simulink model "Full_RC_EVOP"  (Simulink 9.2)
settings: Solver=ode3  StartTime=0.0  StopTime=50000.0  FixedStep=0.01  RelTol=1e-3  EnableMultiTasking=on
settings Model: Creator=user  LastModifiedBy=user
settings DataIOCC: SignalLoggingSaveFormat=Dataset
settings DebuggingCC: UnderspecifiedInitializationDetection=Simplified  MergeDetectMultiDrivingBlocksExec=error  SolverPrmCheckMsg=warning  FcnCallInpInsideContextMsg=error  StateNameClashWarn=none
settings GRTTargetCC: CombineOutputUpdateFcns=on  GRTInterface=off
settings ConfigComp: CovSFcnEnable=off

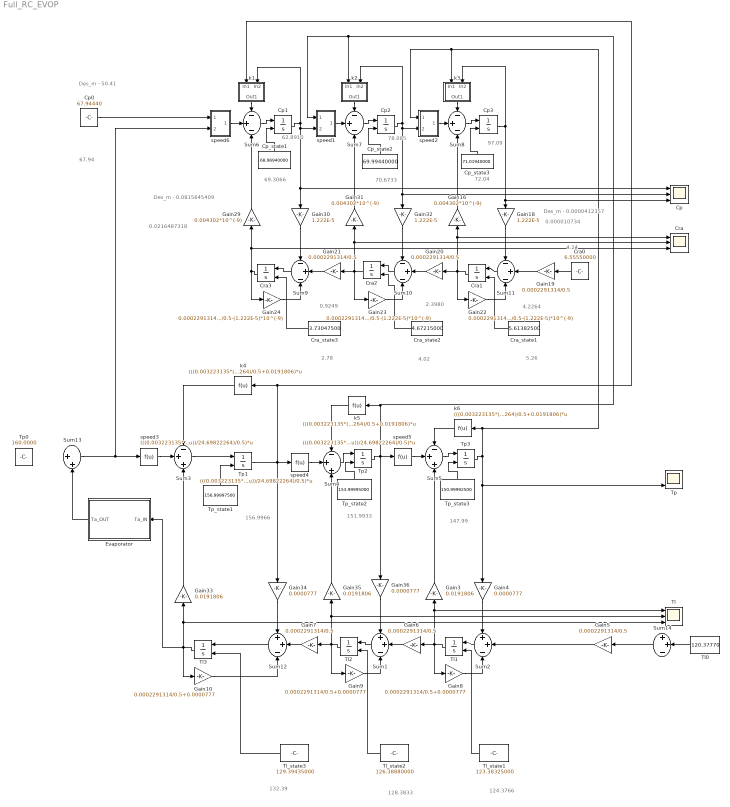
== system Full_RC_EVOP ==
  note: Des_m - 0.0000412357
  note: Des_m - 0.0815645409
  note: 0.000010734
  note: 0.0216487318
  note: 0.9249
  note: 2.3980
  note: 4.2264
  note: 62.8910
  note: 78.085
  note: 97.09
  note: 67.94
  note: 2.78
  note: 4.02
  note: 5.26
  note: 72.04
  note: 70.6733
  note: 69.3066
  note: 132.39
  note: 128.3833
  note: 124.3766
  note: 147.99
  note: 151.9933
  note: 156.9966
  note: 4.24
  note: Des_m - 50.41
  Cp : Scope  NumInputPorts=3
  Cp0 : Constant  Value=67.94440
  Cp1 : Integrator  InitialConditionSource=external  InitialCondition=69.3066
  Cp2 : Integrator  InitialConditionSource=external  InitialCondition=70.6733
  Cp3 : Integrator  InitialConditionSource=external  InitialCondition=72.04
  Cp_state1 : Constant  Value=68.96940000
  Cp_state2 : Constant  Value=69.99440000
  Cp_state3 : Constant  Value=71.01940000
  Cra : Scope  NumInputPorts=3
  Cra0 : Constant  Value=6.55550000
  Cra1 : Integrator  InitialConditionSource=external  InitialCondition=5.26
  Cra2 : Integrator  InitialConditionSource=external  InitialCondition=4.02
  Cra3 : Integrator  InitialConditionSource=external  InitialCondition=2.78
  Cra_state1 : Constant  Value=5.61382500
  Cra_state2 : Constant  Value=4.67215000
  Cra_state3 : Constant  Value=3.73047500
  Evaporator : Subsystem
  Gain10 : Gain  Gain=0.0002291314/0.5+0.0000777
  Gain16 : Gain  Gain=0.004302*10^(-9)
  Gain18 : Gain  Gain=1.222E-5
  Gain{5..7,19..21} (6 alike) : Gain  Gain=0.0002291314/0.5
  Gain22 : Gain  Gain=0.0002291314/0.5-(1.222E-5)*10^(-9)
  Gain23 : Gain  Gain=0.0002291314/0.5-(1.222E-5)*10^(-9)
  Gain24 : Gain  Gain=0.0002291314/0.5-(1.222E-5)*10^(-9)
  Gain29 : Gain  Gain=0.004302*10^(-9)
  Gain3 : Gain  Gain=0.0191806
  Gain30 : Gain  Gain=1.222E-5
  Gain31 : Gain  Gain=0.004302*10^(-9)
  Gain32 : Gain  Gain=1.222E-5
  Gain33 : Gain  Gain=0.0191806
  Gain34 : Gain  Gain=0.0000777
  Gain35 : Gain  Gain=0.0191806
  Gain36 : Gain  Gain=0.0000777
  Gain4 : Gain  Gain=0.0000777
  Gain8 : Gain  Gain=0.0002291314/0.5+0.0000777
  Gain9 : Gain  Gain=0.0002291314/0.5+0.0000777
  Sum{1..2,12,14} (4 alike) : Sum  Inputs=++-
  Sum{6..11} (6 alike) : Sum  Inputs=-+-
  Sum13 : Sum  Inputs=|++
  Sum3 : Sum  Inputs=-++
  Sum4 : Sum  Inputs=-++
  Sum5 : Sum  Inputs=-++
  Tl : Scope  NumInputPorts=3
  Tl0 : Constant  Value=120.37770
  Tl1 : Integrator  InitialConditionSource=external  InitialCondition=124.3766
  Tl2 : Integrator  InitialConditionSource=external  InitialCondition=128.3833
  Tl3 : Integrator  InitialConditionSource=external  InitialCondition=132.39
  "Tl_state1 " : Constant  Value=123.38325000
  Tl_state2 : Constant  Value=126.38880000
  Tl_state3 : Constant  Value=129.39435000
  Tp : Scope  NumInputPorts=3
  Tp0 : Constant  Value=160.0000
  Tp1 : Integrator  InitialConditionSource=external  InitialCondition=156.9966
  Tp2 : Integrator  InitialConditionSource=external  InitialCondition=151.9933
  Tp3 : Integrator  InitialConditionSource=external  InitialCondition=147.99  IgnoreLimit=on
  Tp_state1 : Constant  Value=156.99997500
  Tp_state2 : Constant  Value=153.99995000
  Tp_state3 : Constant  Value=150.99992500
  k1 : Subsystem
  k2 : Subsystem
  k3 : Subsystem
  k4 : Fcn  Expr=(((0.003223135*(273+u))/24.69822264)/0.5+0.0191806)*u
  k5 : Fcn  Expr=(((0.003223135*(273+u))/24.69822264)/0.5+0.0191806)*u
  k6 : Fcn  Expr=(((0.003223135*(273+u))/24.69822264)/0.5+0.0191806)*u
  speed1 : Subsystem
  speed2 : Subsystem
  speed3 : Fcn  Expr=(((0.003223135*(273+u))/24.69822264)/0.5)*u
  speed4 : Fcn  Expr=(((0.003223135*(273+u))/24.69822264)/0.5)*u
  speed5 : Fcn  Expr=(((0.003223135*(273+u))/24.69822264)/0.5)*u
  speed6 : Subsystem
  wires:
  Sum6/1 -> Cp1/1
  speed1/1(Out1) -> Sum7/2
  Sum7/1 -> Cp2/1
  speed2/1(Out1) -> Sum8/2
  Sum8/1 -> Cp3/1
  Cp1/1 -> speed1/2(In2), Gain30/1, Cp/1, k1/2(In2)
  Cp2/1 -> speed2/2(In2), Gain32/1, Cp/2, k2/2(In2)
  Gain29/1 -> Sum6/3
  Cp3/1 -> k3/2(In2), Gain18/1, Cp/3
  Gain31/1 -> Sum7/3
  Gain16/1 -> Sum8/3
  Gain30/1 -> Sum9/1
  Gain32/1 -> Sum10/1
  Gain18/1 -> Sum11/1
  Gain19/1 -> Sum11/2
  Sum11/1 -> Cra1/1
  Cra1/1 -> Gain22/1, Gain20/1, Gain16/1, Cra/1
  Gain20/1 -> Sum10/2
  Sum10/1 -> Cra2/1
  Cra2/1 -> Gain23/1, Gain21/1, Gain31/1, Cra/2
  Gain21/1 -> Sum9/2
  Sum9/1 -> Cra3/1
  Cra3/1 -> Gain24/1, Gain29/1, Cra/3
  Gain22/1 -> Sum11/3
  Gain23/1 -> Sum10/3
  Gain24/1 -> Sum9/3
  speed3/1 -> Sum3/2
  k4/1 -> Sum3/1
  Sum3/1 -> Tp1/1
  speed4/1 -> Sum4/2
  k5/1 -> Sum4/1
  Sum4/1 -> Tp2/1
  speed5/1 -> Sum5/2
  k6/1 -> Sum5/1
  Sum5/1 -> Tp3/1
  Gain33/1 -> Sum3/3
  Tp3/1 -> Gain4/1, Tp/3, k6/1, k3/1(In1), speed2/1(In1)
  Gain35/1 -> Sum4/3
  Gain3/1 -> Sum5/3
  Gain34/1 -> Sum12/1
  Gain36/1 -> Sum1/1
  Gain4/1 -> Sum2/1
  Gain5/1 -> Sum2/2
  Sum2/1 -> Tl1/1
  Tl1/1 -> Gain8/1, Gain6/1, Gain3/1, Tl/1
  Gain6/1 -> Sum1/2
  Sum1/1 -> Tl2/1
  Tl2/1 -> Gain9/1, Gain7/1, Gain35/1, Tl/2
  Gain7/1 -> Sum12/2
  Sum12/1 -> Tl3/1
  Tl3/1 -> Evaporator/1(Ta_IN), Gain10/1, Gain33/1, Tl/3
  Gain8/1 -> Sum2/3
  Gain9/1 -> Sum1/3
  Gain10/1 -> Sum12/3
  speed6/1(Out1) -> Sum6/2
  Cp0/1 -> speed6/1(In1)
  k1/1(Out1) -> Sum6/1
  k2/1(Out1) -> Sum7/1
  k3/1(Out1) -> Sum8/1
  Cra0/1 -> Gain19/1
  Sum13/1 -> speed3/1, speed6/2(In2)
  Sum14/1 -> Gain5/1
  Tl0/1 -> Sum14/2
  Tp2/1 -> Gain36/1, k5/1, speed1/1(In1), k2/1(In1), speed5/1
  Tp1/1 -> k4/1, k1/1(In1), Gain34/1, speed4/1
  Tp_state1/1 -> Tp1/2
  Tp_state2/1 -> Tp2/2
  Tp_state3/1 -> Tp3/2
  "Tl_state1 "/1 -> Tl1/2
  Tl_state2/1 -> Tl2/2
  Tl_state3/1 -> Tl3/2
  Cp_state1/1 -> Cp1/2
  Cp_state2/1 -> Cp2/2
  Cp_state3/1 -> Cp3/2
  Cra_state1/1 -> Cra1/2
  Cra_state2/1 -> Cra2/2
  Cra_state3/1 -> Cra3/2
  Evaporator/1(Ta_OUT) -> Sum13/2

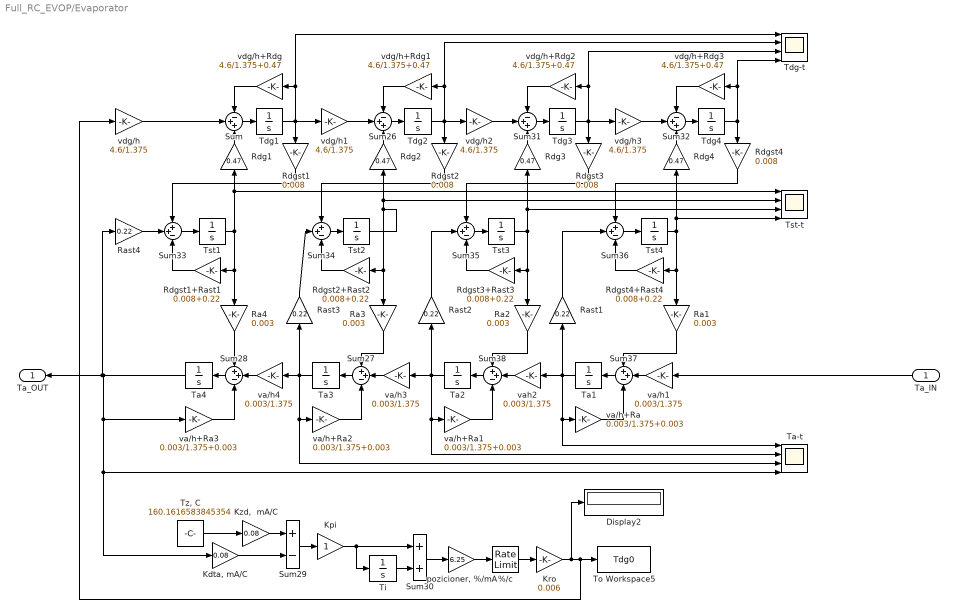
== system Full_RC_EVOP/Evaporator ==
  Ta_IN : Inport
  %/c : RateLimiter  RisingSlewLimit=5  FallingSlewLimit=-5  SampleTimeMode=inherited
  Display2 : Display
  "Kdta, mA/C" : Gain  Gain=0.08
  Kpi : Gain
  Kro : Gain  Gain=0.006
  "Kzd,  mA/C" : Gain  Gain=0.08
  Ra{1..4} (4 alike) : Gain  Gain=0.003
  Rast{1..4} (4 alike) : Gain  Gain=0.22
  Rdg{1..4} (4 alike) : Gain  Gain=0.47
  Rdgst{1..4} (4 alike) : Gain  Gain=0.008
  Rdgst1+Rast1 : Gain  Gain=0.008+0.22
  Rdgst2+Rast2 : Gain  Gain=0.008+0.22
  Rdgst3+Rast3 : Gain  Gain=0.008+0.22
  Rdgst4+Rast4 : Gain  Gain=0.008+0.22
  Sum{,26,31..32} (4 alike) : Sum  Inputs=-++
  Sum{27..28,33..38} (8 alike) : Sum  Inputs=++-
  Sum29 : Sum  Inputs=+-
  Sum30 : Sum
  Ta-t : Scope  NumInputPorts=4
  Ta1 : Integrator  InitialCondition=136.285
  Ta2 : Integrator  InitialCondition=144.19
  Ta3 : Integrator  InitialCondition=152.09
  Ta4 : Integrator  InitialCondition=160
  Tdg-t : Scope  NumInputPorts=4
  Tdg1 : Integrator  InitialCondition=283.3065209436467
  Tdg2 : Integrator  InitialCondition=267.8966165589237
  Tdg3 : Integrator  InitialCondition=253.6715917846216
  Tdg4 : Integrator  InitialCondition=240.5403403000344
  Ti : Integrator  InitialCondition=8000  UpperSaturationLimit=8012  LowerSaturationLimit=6012
  To Workspace5 : ToWorkspace  VariableName=Tdg0  SampleTime=-1
  Tst-t : Scope  NumInputPorts=4
  Tst1 : Integrator  InitialCondition=164.4825307550351
  Tst2 : Integrator  InitialCondition=158.2090959868120
  Tst3 : Integrator  InitialCondition=152.4180305285302
  Tst4 : Integrator  InitialCondition=147.0722446263660
  "Tz, C" : Constant  Value=160.1616583845354
  "pozicioner, %/mA" : Gain  Gain=6.25
  va/h+Ra{,1..3} (4 alike) : Gain  Gain=0.003/1.375+0.003
  va/h1 : Gain  Gain=0.003/1.375
  va/h3 : Gain  Gain=0.003/1.375
  va/h4 : Gain  Gain=0.003/1.375
  vah2 : Gain  Gain=0.003/1.375
  vdg/h{,1..3} (4 alike) : Gain  Gain=4.6/1.375
  vdg/h+Rdg{,1..3} (4 alike) : Gain  Gain=4.6/1.375+0.47
  Ta_OUT : Outport
  wires:
  Sum/1 -> Tdg1/1
  vdg/h2/1 -> Sum31/2
  Sum32/1 -> Tdg4/1
  Tdg2/1 -> vdg/h+Rdg1/1, Tdg-t/2, Rdgst2/1, vdg/h2/1
  Sum26/1 -> Tdg2/1
  vdg/h3/1 -> Sum32/2
  vdg/h/1 -> Sum/2
  Tdg1/1 -> vdg/h+Rdg/1, Tdg-t/1, vdg/h1/1, Rdgst1/1
  vdg/h+Rdg2/1 -> Sum31/1
  vdg/h+Rdg3/1 -> Sum32/1
  Tdg4/1 -> vdg/h+Rdg3/1, Tdg-t/4, Rdgst4/1
  Rdg1/1 -> Sum/3
  Rdg2/1 -> Sum26/3
  Rdg3/1 -> Sum31/3
  Rdg4/1 -> Sum32/3
  vdg/h+Rdg1/1 -> Sum26/1
  Sum33/1 -> Tst1/1
  Sum34/1 -> Tst2/1
  Tdg3/1 -> vdg/h+Rdg2/1, Tdg-t/3, vdg/h3/1, Rdgst3/1
  vdg/h1/1 -> Sum26/2
  Sum35/1 -> Tst3/1
  vdg/h+Rdg/1 -> Sum/1
  Sum31/1 -> Tdg3/1
  Rdgst3+Rast3/1 -> Sum35/3
  Tst1/1 -> Rdgst1+Rast1/1, Ra4/1, Rdg1/1, Tst-t/1
  Rdgst1+Rast1/1 -> Sum33/3
  Tst3/1 -> Rdgst3+Rast3/1, Ra2/1, Rdg3/1, Tst-t/3
  Tst2/1 -> Rdg2/1, Tst-t/2, Rdgst2+Rast2/1, Ra3/1
  Rdgst1/1 -> Sum33/1
  Rdgst2/1 -> Sum34/1
  Tst4/1 -> Rdgst4+Rast4/1, Ra1/1, Rdg4/1, Tst-t/4
  Rdgst4/1 -> Sum36/1
  Rdgst2+Rast2/1 -> Sum34/3
  va/h1/1 -> Sum37/2
  va/h+Ra/1 -> Sum37/3
  Rdgst3/1 -> Sum35/1
  Sum36/1 -> Tst4/1
  Rdgst4+Rast4/1 -> Sum36/3
  Ti/1 -> Sum30/2
  Ta4/1 -> Ta_OUT/1, Rast4/1, va/h+Ra3/1, Ta-t/4, "Kdta, mA/C"/1
  Rast1/1 -> Sum36/2
  Ra2/1 -> Sum38/1
  Ta2/1 -> va/h+Ra1/1, Ta-t/2, va/h3/1, Rast2/1
  va/h+Ra3/1 -> Sum28/3
  Ta1/1 -> Ta-t/1, va/h+Ra/1, Rast1/1, vah2/1
  va/h+Ra2/1 -> Sum27/3
  Rast3/1 -> Sum34/2
  Sum38/1 -> Ta2/1
  va/h4/1 -> Sum28/2
  Sum37/1 -> Ta1/1
  va/h3/1 -> Sum27/2
  Ta3/1 -> va/h+Ra2/1, Ta-t/3, va/h4/1, Rast3/1
  Rast2/1 -> Sum35/2
  "Tz, C"/1 -> "Kzd,  mA/C"/1
  "Kdta, mA/C"/1 -> Sum29/2
  %/c/1 -> Kro/1
  Ta_IN/1 -> va/h1/1
  "Kzd,  mA/C"/1 -> Sum29/1
  Sum28/1 -> Ta4/1
  Rast4/1 -> Sum33/2
  Sum27/1 -> Ta3/1
  va/h+Ra1/1 -> Sum38/3
  "pozicioner, %/mA"/1 -> %/c/1
  Ra3/1 -> Sum27/1
  Sum29/1 -> Kpi/1
  Kpi/1 -> Sum30/1, Ti/1
  Ra4/1 -> Sum28/1
  Sum30/1 -> "pozicioner, %/mA"/1
  Kro/1 -> To Workspace5/1, vdg/h/1, Display2/1
  Ra1/1 -> Sum37/1
  vah2/1 -> Sum38/2

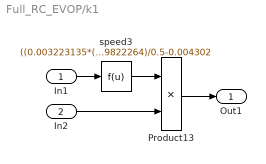
== system Full_RC_EVOP/k1 ==
  In1 : Inport
  In2 : Inport  Port=2
  Product13 : Product  SaturateOnIntegerOverflow=on  InputSameDT=on  OutDataTypeStr=Inherit: Same as first input
  speed3 : Fcn  Expr=((0.003223135*(273+u))/24.69822264)/0.5-0.004302
  Out1 : Outport
  wires:
  Product13/1 -> Out1/1
  speed3/1 -> Product13/1
  In1/1 -> speed3/1
  In2/1 -> Product13/2

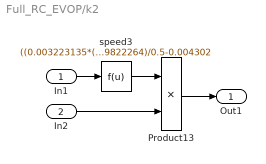
== system Full_RC_EVOP/k2 ==
  In1 : Inport
  In2 : Inport  Port=2
  Product13 : Product  SaturateOnIntegerOverflow=on  InputSameDT=on  OutDataTypeStr=Inherit: Same as first input
  speed3 : Fcn  Expr=((0.003223135*(273+u))/24.69822264)/0.5-0.004302
  Out1 : Outport
  wires:
  Product13/1 -> Out1/1
  speed3/1 -> Product13/1
  In1/1 -> speed3/1
  In2/1 -> Product13/2

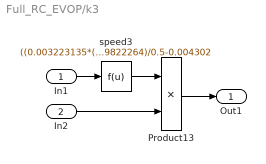
== system Full_RC_EVOP/k3 ==
  In1 : Inport
  In2 : Inport  Port=2
  Product13 : Product  SaturateOnIntegerOverflow=on  InputSameDT=on  OutDataTypeStr=Inherit: Same as first input
  speed3 : Fcn  Expr=((0.003223135*(273+u))/24.69822264)/0.5-0.004302
  Out1 : Outport
  wires:
  Product13/1 -> Out1/1
  speed3/1 -> Product13/1
  In1/1 -> speed3/1
  In2/1 -> Product13/2

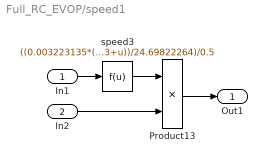
== system Full_RC_EVOP/speed1 ==
  In1 : Inport
  In2 : Inport  Port=2
  Product13 : Product  SaturateOnIntegerOverflow=on  InputSameDT=on  OutDataTypeStr=Inherit: Same as first input
  speed3 : Fcn  Expr=((0.003223135*(273+u))/24.69822264)/0.5
  Out1 : Outport
  wires:
  Product13/1 -> Out1/1
  In2/1 -> Product13/2
  speed3/1 -> Product13/1
  In1/1 -> speed3/1

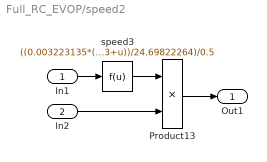
== system Full_RC_EVOP/speed2 ==
  In1 : Inport
  In2 : Inport  Port=2
  Product13 : Product  SaturateOnIntegerOverflow=on  InputSameDT=on  OutDataTypeStr=Inherit: Same as first input
  speed3 : Fcn  Expr=((0.003223135*(273+u))/24.69822264)/0.5
  Out1 : Outport
  wires:
  Product13/1 -> Out1/1
  In2/1 -> Product13/2
  speed3/1 -> Product13/1
  In1/1 -> speed3/1

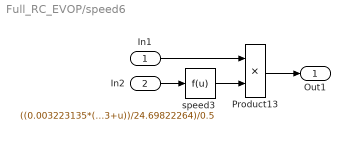
== system Full_RC_EVOP/speed6 ==
  In1 : Inport
  In2 : Inport  Port=2
  Product13 : Product  SaturateOnIntegerOverflow=on  InputSameDT=on  OutDataTypeStr=Inherit: Same as first input
  speed3 : Fcn  Expr=((0.003223135*(273+u))/24.69822264)/0.5
  Out1 : Outport
  wires:
  In1/1 -> Product13/1
  In2/1 -> speed3/1
  speed3/1 -> Product13/2
  Product13/1 -> Out1/1
